simulink model "ljabos"  (Simulink 6.5)
settings: Solver=ode45  StartTime=0.0  StopTime=100000  RelTol=1e-3
settings Model: Creator=rr44526  LastModifiedBy=rr44526

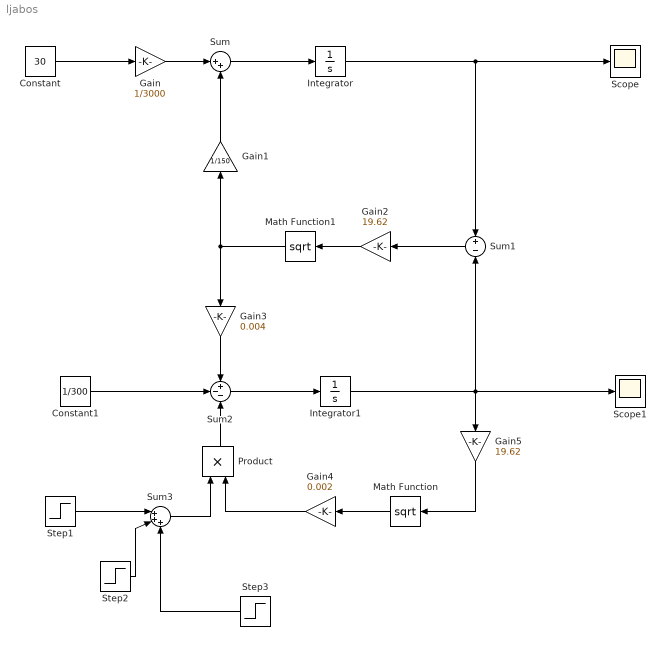
== system ljabos ==
  Constant : Constant  Value=30  OutDataType=sfix(16)  ConRadixGroup=Use specified scaling  OutScaling=2^0  SampleTime=inf  FramePeriod=inf
  Constant1 : Constant  Value=1/300  OutDataType=sfix(16)  ConRadixGroup=Use specified scaling  OutScaling=2^0  SampleTime=inf  FramePeriod=inf
  Gain : Gain  Gain=1/3000
  Gain1 : Gain  Orientation=up  Gain=1/150
  Gain2 : Gain  Orientation=left  Gain=19.62
  Gain3 : Gain  Orientation=down  Gain=0.004
  Gain4 : Gain  Orientation=left  Gain=0.002
  Gain5 : Gain  Orientation=down  Gain=19.62
  Integrator : Integrator  LimitOutput=on  UpperSaturationLimit=10  LowerSaturationLimit=0
  Integrator1 : Integrator  LimitOutput=on  UpperSaturationLimit=10  LowerSaturationLimit=0
  Math Function : Math  Orientation=left  Operator=sqrt  SaturateOnIntegerOverflow=on
  Math Function1 : Math  Orientation=left  Operator=sqrt  SaturateOnIntegerOverflow=on
  Product : Product  Orientation=up  RndMeth=Zero
  Scope : Scope
      settings: TimeRange=100000  YMin=0  YMax=10
  Scope1 : Scope
      settings: TimeRange=1000  YMin=0  YMax=10
  Step1 : Step  Time=0  After=0.3  SampleTime=0
  Step2 : Step  Time=20000  After=0.06  SampleTime=0
  Step3 : Step  Orientation=left  Time=40000  After=-0.12  SampleTime=0
  Sum : Sum  Inputs=|++
  Sum1 : Sum  Orientation=left  Inputs=+-
  Sum2 : Sum  Inputs=+--
  Sum3 : Sum  Inputs=|+++
  wires:
  Constant/1 -> Gain/1
  Gain/1 -> Sum/1
  Gain1/1 -> Sum/2
  Sum/1 -> Integrator/1
  Integrator/1 -> Scope/1, Sum1/1
  Sum1/1 -> Gain2/1
  Gain2/1 -> Math Function1/1
  Math Function1/1 -> Gain3/1, Gain1/1
  Gain3/1 -> Sum2/1
  Sum2/1 -> Integrator1/1
  Integrator1/1 -> Scope1/1, Sum1/2, Gain5/1
  Gain5/1 -> Math Function/1
  Math Function/1 -> Gain4/1
  Gain4/1 -> Product/2
  Product/1 -> Sum2/3
  Constant1/1 -> Sum2/2
  Sum3/1 -> Product/1
  Step1/1 -> Sum3/1
  Step3/1 -> Sum3/3
  Step2/1 -> Sum3/2
